simulink model "test_trajGen"  (R2017b)
settings: Solver=VariableStepAuto  StartTime=0.0  StopTime=20  RelTol=1e-3
settings Model: Creator=chao  LastModifiedBy=chao

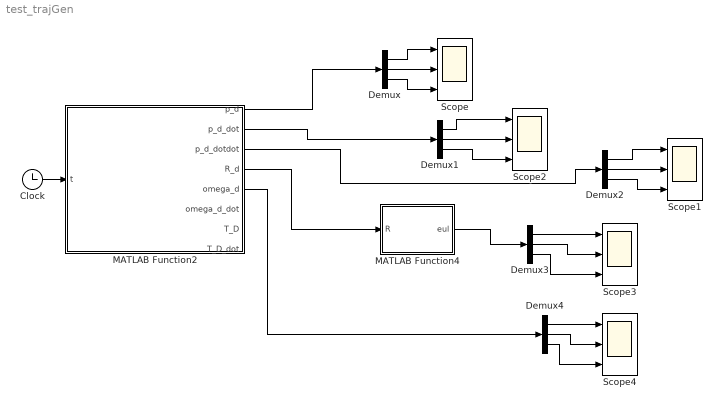
== system test_trajGen ==
  Clock : Clock
  Demux{,1..4} (5 alike) : Demux  Outputs=3
  MATLAB Function2 : MATLAB Function  TreatAsAtomicUnit=on
  MATLAB Function4 : MATLAB Function  TreatAsAtomicUnit=on
  Scope{,1..4} (5 alike) : Scope  NumInputPorts=3
  wires:
  Clock/1 -> MATLAB Function2/1(t)
  MATLAB Function2/1(p_d) -> Demux/1
  Demux/1 -> Scope/1
  Demux/2 -> Scope/2
  Demux/3 -> Scope/3
  MATLAB Function2/2(p_d_dot) -> Demux1/1
  Demux1/1 -> Scope2/1
  Demux1/2 -> Scope2/2
  Demux1/3 -> Scope2/3
  MATLAB Function2/3(p_d_dotdot) -> Demux2/1
  Demux2/1 -> Scope1/1
  Demux2/2 -> Scope1/2
  Demux2/3 -> Scope1/3
  MATLAB Function2/4(R_d) -> MATLAB Function4/1(R)
  MATLAB Function4/1(eul) -> Demux3/1
  Demux3/1 -> Scope3/1
  Demux3/2 -> Scope3/2
  Demux3/3 -> Scope3/3
  Demux4/1 -> Scope4/1
  Demux4/2 -> Scope4/2
  Demux4/3 -> Scope4/3
  MATLAB Function2/5(omega_d) -> Demux4/1

== matlab function test_trajGen/MATLAB Function4 ==
  data: R input; eul output
function eul = DCM2Euler(R)

%Roll
phi = atan2d(R(3,2),R(3,3));

%Pitch
psi = atan2d(-R(3,1),sqrt(R(1,1)^2 + R(2,1)^2));

%Yaw
gamma = atan2d(R(2,1),R(1,1));

eul=[phi;psi;gamma];

== matlab function test_trajGen/MATLAB Function2 ==
  data: t input; p_d output; p_d_dot output; p_d_dotdot output; R_d output; omega_d output; omega_d_dot output; T_D output; T_D_dot output
function [p_d, p_d_dot, p_d_dotdot, R_d, omega_d, omega_d_dot, T_D, T_D_dot] = createTrajectory(t)

if t < 10
    %zeros
    % 
    p_d = [0;0;0];
    p_d_dot = [0;0;0];
    p_d_dotdot = [0;0;0];
    R_d = eye(3);
    omega_d = [0;0;0];
    omega_d_dot = [0;0;0];
    T_D = zeros(6,1);
    T_D_dot = zeros(6,1);

else
%     p_d = [1;0.75;0.5];
%     p_d_dot = [0;0;0];
%     p_d_dotdot = [0;0;0];
%     
%     ct = cosd(10); % roll
%     st = sind(10);
%     ct2 = cosd(7.5); % pitch
%     st2 = sind(7.5);
%     ct3 = cosd(15); % yaw
%     st3 = sind(15);
%     R_d = [ct3, -st3, 0; 
%             st3, ct3, 0;
%             0, 0, 1]*[ct2, 0, st2; 
%             0, 1, 0;
%             -st2, 0, ct2]*[1 0 0;
%             0 ct, -st; 
%            0 st, ct];
%     omega_d = [0;0;0];
%     omega_d_dot = [0;0;0];
%     T_D = zeros(6,1);
%     T_D_dot = zeros(6,1);
%     
    
        t = t-10;
    xa = 0;
    xe = 0.5;
    te = 5;
    x = xa + 10*(xe-xa)*t^3/te^3 - 15*(xe-xa)*t^4/te^4 + 6*(xe-xa)*t^5/te^5;
    x_dot = 3*10*(xe-xa)*t^2/te^3 - 4*15*(xe-xa)*t^3/te^4 + 5*6*(xe-xa)*t^4/te^5;
    x_dot_dot = 6*10*(xe-xa)*t/te^3 - 12*15*(xe-xa)*t^2/te^4 + 20*6*(xe-xa)*t^3/te^5;
    if (t> te)
        x = xe;
        x_dot = 0;
        x_dot_dot = 0;
    end
    p_d = [x;0;x];
    p_d_dot = [x_dot;0;x_dot];
    p_d_dotdot = [x_dot_dot;0;x_dot_dot];
    
    xe = 1;
    x = xa + 10*(xe-xa)*t^3/te^3 - 15*(xe-xa)*t^4/te^4 + 6*(xe-xa)*t^5/te^5;
    x_dot = 3*10*(xe-xa)*t^2/te^3 - 4*15*(xe-xa)*t^3/te^4 + 5*6*(xe-xa)*t^4/te^5;
    x_dot_dot = 6*10*(xe-xa)*t/te^3 - 12*15*(xe-xa)*t^2/te^4 + 20*6*(xe-xa)*t^3/te^5;
    if (t> te)
        x = xe;
        x_dot = 0;
        x_dot_dot = 0;
    end
    p_d(3) = x;
    p_d_dot(3) = x_dot;
    p_d_dotdot(3) = x_dot_dot;
    
    yaw_e = 2*pi/3;
    a = yaw_e/te;
    ct = cos(a*t);
    st = sin(a*t);
    
    R_d = [ct, -st, 0; 
           st, ct, 0;
           0 0 1];
    R_d_dot = [-a*st, -a*ct, 0;
                a*ct, -a*st, 0;
                0 0 0];
    R_d_dotdot = [-a*a*ct, a*a*st, 0;
                   -a*a*st, -a*a*ct, 0;
                   0 0 0];
               
    T_d_tilde = [R_d', -R_d'*p_d; 0,0,0,1]*[R_d_dot p_d_dot; 0,0,0,0];
    
    omega_d = skew2vec(T_d_tilde(1:3,1:3));
    
    T_d_tilde_dot = [R_d_dot'*R_d_dot+R_d'*R_d_dotdot, R_d_dot'*p_d_dot+R_d'*p_d_dotdot;
        0,0,0,0];
    
    omega_d_dot = skew2vec(T_d_tilde_dot(1:3,1:3));
    
    T_D = [omega_d; T_d_tilde(1:3,4)];
    T_D_dot = [omega_d_dot; T_d_tilde_dot(1:3,4)];
    
    if t>te
        R_d = [cos(yaw_e), -sin(yaw_e), 0; 
           sin(yaw_e), cos(yaw_e), 0;
           0 0 1];
        omega_d = [0;0;0];
        omega_d_dot = [0;0;0];
        T_D = zeros(6,1);
        T_D_dot = zeros(6,1);
    end
end

%     p_d = [0;0;0];
%     p_d_dot = [0;0;0];
%     p_d_dotdot = [0;0;0];
%     R_d = eye(3);
%     omega_d = [0;0;0];
%     omega_d_dot = [0;0;0];
%     T_D = zeros(6,1);
%     T_D_dot = zeros(6,1);
end
